simulink library "xbsIndex_r4"  (Simulink 7.1)
PreLoadFcn:
  | warning('off','MATLAB:mex:deprecatedExtension');xlmeta;com.xilinx.sysgen.util.StrategyUtil.loadAllStrategyNames();
values from neighbouring files (symbols this model uses):
  a = xpath.evaluate('//pre:DocumentInfo/pre:Document',x,javax.xml.xpath.XPathConstants.NODESET)    [xlDoc.m]
  n = xpath.evaluate(['//pre:DocumentInfo/pre:Document[@title="'  title                            '"]'],root_elem,javax.xml.xpath.XPathConstants.NODE)    [xlDoc.m]
undefined symbols (not defined in the file or in its folder): gcbh, sim_pause, simulink_period, xlBlockLoadCallback, xlipgetpartsetting, xlRegisterHandles, xlUpdateSgTokenIconStats
libraries: xbsIndex_r4 x18, xbsCopyrightNotice_r4 x1, simulink x1
(part 9 of 9)

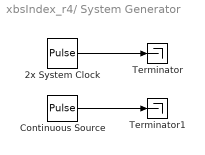
== system xbsIndex_r4/ System Generator ==
  2x System Clock : DiscretePulseGenerator  SampleTime=simulink_period
  Continuous Source : DiscretePulseGenerator  PulseType=Time based  Period=2*simulink_period  PulseWidth=50
  Terminator : Terminator
  Terminator1 : Terminator
  wires:
  Continuous Source/1 -> Terminator1/1
  2x System Clock/1 -> Terminator/1

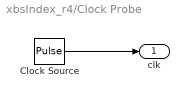
== system xbsIndex_r4/Clock Probe ==
  Clock Source : DiscretePulseGenerator  PhaseDelay=2  SampleTime=(simulink_period/2)
  clk : Outport  OutDataType=sfix(16)  OutScaling=2^0
  wires:
  Clock Source/1 -> clk/1

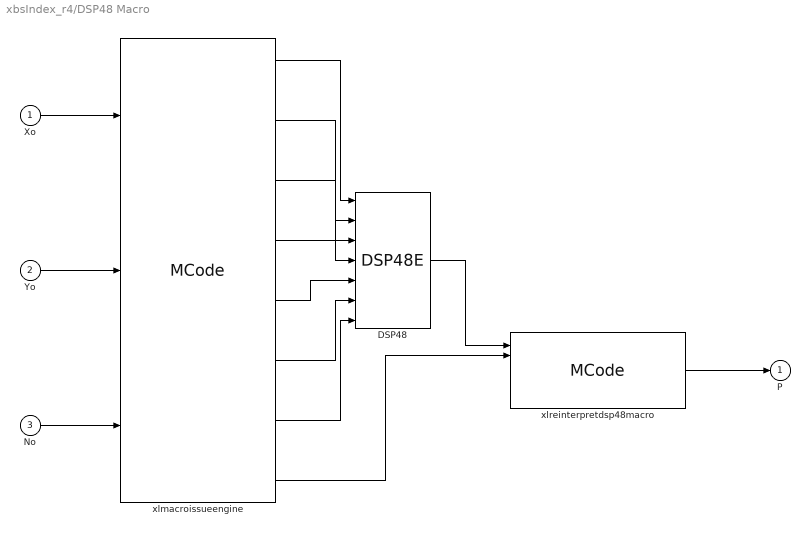
== system xbsIndex_r4/DSP48 Macro ==
  Xo : Inport  OutDataType=sfix(16)  OutScaling=2^0
  Yo : Inport  Port=2  OutDataType=sfix(16)  OutScaling=2^0
  No : Inport  Port=3  OutDataType=sfix(16)  OutScaling=2^0
  DSP48 : xbsIndex_r4/DSP48E  use_a=Direct from A Port  use_b=Direct from B Port  reset_preg=off  pattern_from_creg=on  pattern='000000000000'  mask_from_creg=on  pattern_mask='000000000000'  sel_rounding_mask=Select mask  use_op=off  use_creg=on  rst_all=off  en_all=off  use_pcin=off  use_carrycascin=off  use_multsignin=off  use_carryout=off  use_patterndetect=off  use_patternbdetect=off  use_overflow=off  use_underflow=off  use_acout=off  use_bcout=off  use_pcout=off  use_multsignout=off  use_carrycascout=off  pipeline_a=1  pipeline_b=1  pipeline_acout=1  pipeline_bcout=1  pipeline_c=on  pipeline_p=on  pipeline_mult=on  pipeline_opmode=on  pipeline_alumode=on  pipeline_carryin=on  pipeline_carryinsel=on  rst_a=off  rst_b=off  rst_c=off  rst_mult=off  rst_p=off  rst_carry_in=off  rst_alumode=off  rst_ctrl=off  en_a1=off  en_a2=off  en_b1=off  en_b2=off  en_c=off  en_mult=off  en_p=off  en_carry_in=off  en_alumode=off  en_multcarryin=off  en_ctrl=off  use_synth_model=off  addsub_mode=ONE48  xl_useadderonly=off  block_type=dsp48e
  xlmacroissueengine : xbsIndex_r4/MCode  mfname=xlissue_engine_v5  explicit_period=off  period=1  dbl_ovrd=off  enable_stdout=off  enable_debug=off  suppress_output=on  defparams={'id_a1', 0,'id_a2', 0,'id_a3', 0,'id_a4', 0,'id_a5', 0,'id_a6', 0,'id_a7', 0,'id_b1', 0,'id_b2', 0,'id_b3', 0,'id_b4', 0,'id_b5', 0,'id_b6', 0,'id_b7', 0,'id_c1', 0,'id_c2', 0,'id_c3', 0,'id_c4', 0,'id_c5', 0,'id_c6', 0,'id_c7', 0,'op_const0',53,'op_const1', 0,'op_const2', 0,'op_const3', 0,'op_const4', 0,'op_const5', 0,'op_const6', 0,'op_const7', 0,'alumode_const0',0,'alumode_const1', 0,'alumode_const2', 0,'alumode_const3', 0,'alumode_const4', 0,'alumode_const5', 0,'alumode_const6', 0,'alumode_const7', 0,'carry_in_sel0',0,'carry_in_sel1', 0,'carry_in_sel2', 0,'carry_in_sel3', 0,'carry_in_sel4', 0,'carry_in_sel5', 0,'carry_in_sel6', 0,'carry_in_sel7', 0,'external_cin0', 0,'external_cin1', 0,'external_cin2', 0,'external_cin3', 0,'external_cin4', 0,'external_cin5', 0,'external_cin6', 0,'external_cin7', 0,'reg_a',0,'reg_b',0,'reg_c',0,'reg_op',0,'mode0', 1,'mode1', 0,'mode2', 0,'mode3', 0,'mode4', 0,'mode5', 0,'mode6', 0,'mode7', 0,'ce_all',true,'use_ce_all',false,'sel',0,'rst_all',false,'use_rst_all',false,'cinused',false,'ninstr',1}  hide_port_list={}  block_type=mcode
      settings: xl_area=[0, 0, 0, 0, 0, 0, 0]
  xlreinterpretdsp48macro : xbsIndex_r4/MCode  mfname=xlreinterpretdsp48macro  explicit_period=off  period=1  dbl_ovrd=off  enable_stdout=off  enable_debug=off  suppress_output=off  defparams={'full',precision,'n_bits',n_bits,'bin_pt',bin_pt,'arith_type',arith_type}  hide_port_list={}  block_type=mcode
      settings: xl_area=[0, 0, 0, 0, 0, 0, 0]
  P : Outport  OutDataType=sfix(16)  OutScaling=2^0
  wires:
  xlreinterpretdsp48macro/1 -> P/1
  DSP48/1 -> xlreinterpretdsp48macro/1
  xlmacroissueengine/8 -> xlreinterpretdsp48macro/2
  xlmacroissueengine/7 -> DSP48/7
  xlmacroissueengine/6 -> DSP48/6
  xlmacroissueengine/5 -> DSP48/5
  xlmacroissueengine/4 -> DSP48/4
  xlmacroissueengine/3 -> DSP48/3
  xlmacroissueengine/2 -> DSP48/2
  xlmacroissueengine/1 -> DSP48/1
  No/1 -> xlmacroissueengine/3
  Yo/1 -> xlmacroissueengine/2
  Xo/1 -> xlmacroissueengine/1

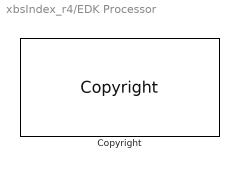
== system xbsIndex_r4/EDK Processor ==
  Copyright : xbsCopyrightNotice_r4/Copyright  copyrighttext="Copyright (c) 2011  by  Xilinx, Inc. All rights reserved.<br><br>This file contains proprietary, confidential information of Xilinx, Inc., is distributed under license from Xilinx, Inc., and may be used, copied and/or disclosed only pursuant to the terms of a valid license agreement with Xilinx, Inc. Xilinx hereby grants you a license to use this file solely for design, simulation, implementation and creation of design files limited to Xilinx devices or technologies. Use with non-Xilinx devices or technologies is expressly prohibited and immediately terminates your license unless covered by a separate agreement.<br><br>Xilinx is providing this design, code, or information \"as-is\" solely for use in developing programs and solutions for Xilinx devices, with no obligation on the part of Xilinx to provide support. By providing this design, code, or information as one possible implementation of this feature, application or standard, Xilinx is making no representation that this implementation is free from any claims of infringement. You are responsible for obtaining any rights you may require for your implementation. Xilinx expressly disclaims any warranty whatsoever with respect to the adequacy of the implementation, including but not limited to any warranties or representations that this implementation is free from claims of infringement, implied warranties of merchantability or fitness for a particular purpose.<br><br>Xilinx products are not intended for use in life support appliances, devices, or systems. Use in such applications is expressly prohibited.<br><br>Any modifications that are made to the Source Code are done at the user's sole risk and will be unsupported.<br><br>This copyright and support notice must be retained as part of this text at all times. (c) Copyright 1995-2011 Xilinx, Inc. All rights reserved."  block_type=copyright
      settings: block_version=10.1.3
      settings: infoedit=|
      | Copyright(C) 2008 by  Xilinx, Inc. All rights reserved.<br>
      | <br>
      | This file contains proprietary, confidential information of Xilinx, Inc., is distributed under license
      | from Xilinx, Inc., and may be used, copied and/or disclosed only pursuant to the terms of a valid license
      | agreement with Xilinx, Inc. Xilinx hereby grants you a license to use this file solely for design,
      | simulation, implementation and creation of design files limited to Xilinx devices or technologies. Use
      | with non-Xilinx devices or technologies is expressly prohibited and immediately terminates your license
      | unless covered by a separate agreement.<br>
      | <br>
      | Xilinx is providing this design, code, or information "as-is" solely for use in developing programs and
      | solutions for Xilinx devices, with no obligation on the part of Xilinx to provide support. By providing
      | this design, code, or information as one possible implementation of this feature, application or standard,
      | Xilinx is making no representation that this implementation is free from any claims of infringement. You
      | are responsible for obtaining any rights you may require for your implementation. Xilinx expressly disclaims
      | any warranty whatsoever with respect to the adequacy of the implementation, including but not limited to any
      | warranties or representations that this implementation is free from claims of infringement, implied warranties
      | of merchantability or fitness for a particular purpose.<br>
      | <br>
      | Xilinx products are not intended for use in life support appliances, devices, or systems. Use in such
      | applications is expressly prohibited.<br>
      | <br>
      | Any modifications that are made to the Source Code are done at the user's sole risk and will be unsupported.<br>
      | <br>
      | This copyright and support notice must be retained as part of this text at all times.
      | (c) Copyright 1995-2008 Xilinx, Inc. All rights reserved.

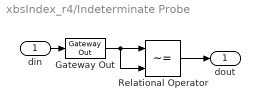
== system xbsIndex_r4/Indeterminate Probe ==
  din : Inport  OutDataType=sfix(16)  OutScaling=2^0
  Gateway Out : xbsIndex_r4/Gateway Out  inherit_from_input=off  hdl_port=off  timing_constraint=None  locs_specified=off  LOCs={}  UseAsDAC=off  DACChannel='1'  block_type=gatewayout
      settings: infoedit="Gateway out block.  Converts Xilinx fixed point inputs into ouputs of type Simulink integer, double, or fixed point.<P><P>Hardware notes:  In hardware these blocks become top level output ports or are discarded, depending on how they are configured."  block_version=9.2-dev
  Relational Operator : RelationalOperator  Operator=~=  InputSameDT=on
  dout : Outport  OutDataType=sfix(16)  OutScaling=2^0
  wires:
  Gateway Out/1 -> Relational Operator/1, Relational Operator/2
  Relational Operator/1 -> dout/1
  din/1 -> Gateway Out/1

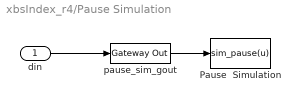
== system xbsIndex_r4/Pause Simulation ==
  din : Inport  OutDataType=sfix(16)  OutScaling=2^0
  Pause  Simulation : MATLABFcn  Priority=1000  MATLABFcn=sim_pause(u)  OutputDimensions=0  Output1D=off
  pause_sim_gout : xbsIndex_r4/Gateway Out  inherit_from_input=off  hdl_port=off  timing_constraint=None  locs_specified=off  LOCs={}  UseAsDAC=off  DACChannel='1'  block_type=gatewayout
      settings: infoedit="Gateway out block.  Converts Xilinx fixed point inputs into ouputs of type Simulink integer, double, or fixed point.<br><br>Hardware notes:  In hardware these blocks become top level output ports or are discarded, depending on how they are configured."  block_version=11.3
  wires:
  pause_sim_gout/1 -> Pause  Simulation/1
  din/1 -> pause_sim_gout/1

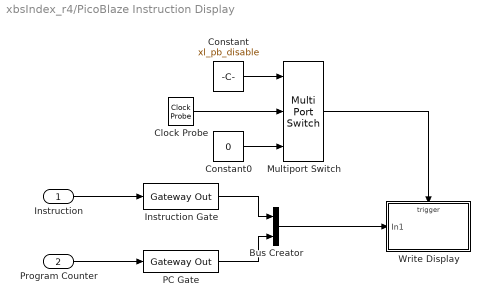
== system xbsIndex_r4/PicoBlaze Instruction Display ==
  Instruction : Inport  OutDataType=sfix(16)  OutScaling=2^0
  Program Counter : Inport  Port=2  OutDataType=sfix(16)  OutScaling=2^0
  Bus Creator : BusCreator  Inputs=2
  Clock Probe : xbsIndex_r4/Clock Probe  SystemSampleTime=-1  block_type=clkprobe
      settings: infoedit="Clock probe.  Produces an output of type double that mirrors the hardware system clock.<P><P>Hardware notes:  This block is ignored when hardware is generated."  block_version=9.1-dev2
  Constant : Constant  Value=xl_pb_disable  OutDataType=sfix(16)  OutScaling=2^0
  Constant0 : Constant  Value=0  OutDataType=sfix(16)  OutScaling=2^0
  Instruction Gate : xbsIndex_r4/Gateway Out  inherit_from_input=off  hdl_port=off  timing_constraint=None  locs_specified=off  LOCs={}  UseAsDAC=off  DACChannel='1'  block_type=gatewayout
      settings: infoedit="Gateway out block.  Converts Xilinx fixed point inputs into ouputs of type Simulink integer, double, or fixed point.<P><P>Hardware notes:  In hardware these blocks become top level output ports or are discarded, depending on how they are configured."  xl_area=[0, 0, 0, 0, 0, 0, 0]  block_version=9.1-dev2
  Multiport Switch : MultiPortSwitch  Inputs=2  zeroidx=on  SaturateOnIntegerOverflow=on
  PC Gate : xbsIndex_r4/Gateway Out  inherit_from_input=off  hdl_port=off  timing_constraint=None  locs_specified=off  LOCs={}  UseAsDAC=off  DACChannel='1'  block_type=gatewayout
      settings: infoedit="Gateway out block.  Converts Xilinx fixed point inputs into ouputs of type Simulink integer, double, or fixed point.<P><P>Hardware notes:  In hardware these blocks become top level output ports or are discarded, depending on how they are configured."  xl_area=[0, 0, 0, 0, 0, 0, 0]  block_version=9.1-dev2
  Write Display : Subsystem  AncestorBlock=xbsIndex_r4/PicoBlaze Instruction Display/Write Display  mask{xl_pb_inst=LOAD sC, 12, xl_pb_pc=17, xl_pb_version=xl_pb_version}
      mask prompts: xl_pb_version "PicoBlaze Version"
  wires:
  Constant0/1 -> Multiport Switch/3
  Clock Probe/1 -> Multiport Switch/2
  Multiport Switch/1 -> Write Display/Trigger
  Constant/1 -> Multiport Switch/1
  Instruction/1 -> Instruction Gate/1
  Program Counter/1 -> PC Gate/1
  Instruction Gate/1 -> Bus Creator/1
  PC Gate/1 -> Bus Creator/2
  Bus Creator/1 -> Write Display/1(In1)

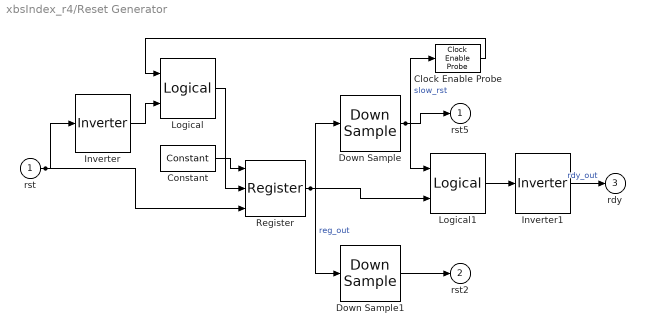
== system xbsIndex_r4/Reset Generator ==
  rst : Inport
  Clock Enable Probe : xbsIndex_r4/Clock Enable Probe  inherit_constraints=on  block_type=ceprobe
      settings: infoedit="Clock enable extractor.  Produces a Boolean output that mirrors the hardware clock enable associated with the input sample rate.<br><br>Hardware notes: in hardware this block costs nothing."
  Constant : xbsIndex_r4/Constant  const=1  gui_display_data_type=Fixed-point  arith_type=Boolean  n_bits=1  bin_pt=0  preci_type=Single  exp_width=8  frac_width=24  explicit_period=off  period=1  equ=P=C  opselect=C  inp2=PCIN>>17  opr=+  inp1=P  carry=CIN  dbl_ovrd=off  block_type=constant
  Down Sample : xbsIndex_r4/Down Sample  sample_ratio=5  sample_phase="Last Value of Frame  (most efficient)"  en=off  latency=1  dbl_ovrd=off  block_type=dsamp
  Down Sample1 : xbsIndex_r4/Down Sample  sample_ratio=2  sample_phase="Last Value of Frame  (most efficient)"  en=off  latency=3  dbl_ovrd=off  block_type=dsamp
  Inverter : xbsIndex_r4/Inverter  en=off  latency=0  dbl_ovrd=off  block_type=inv
  Inverter1 : xbsIndex_r4/Inverter  en=off  latency=0  dbl_ovrd=off  block_type=inv
  Logical : xbsIndex_r4/Logical  logical_function=AND  inputs=2  en=off  latency=0  precision=Full  arith_type=Unsigned  n_bits=16  bin_pt=0  align_bp=on  dbl_ovrd=off  block_type=logical
  Logical1 : xbsIndex_r4/Logical  logical_function=OR  inputs=2  en=off  latency=0  precision=Full  arith_type=Unsigned  n_bits=16  bin_pt=0  align_bp=on  dbl_ovrd=off  block_type=logical
  Register : xbsIndex_r4/Register  init=0  rst=on  en=on  dbl_ovrd=off  block_type=register
  rst5 : Outport
  rst2 : Outport  Port=2
  rdy : Outport  Port=3
  wires:
  Down Sample/1 -> rst5/1, Logical1/1, Clock Enable Probe/1  "slow_rst"
  rst/1 -> Register/3, Inverter/1
  Register/1 -> Down Sample1/1, Logical1/2, Down Sample/1  "reg_out"
  Inverter1/1 -> rdy/1  "rdy_out"
  Down Sample1/1 -> rst2/1
  Logical1/1 -> Inverter1/1
  Logical/1 -> Register/2
  Constant/1 -> Register/1
  Inverter/1 -> Logical/2
  Clock Enable Probe/1 -> Logical/1

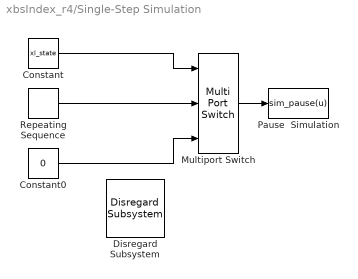
== system xbsIndex_r4/Single-Step Simulation ==
  Constant : Constant  Value=xl_state  OutDataType=sfix(16)  OutScaling=2^0
  Constant0 : Constant  Value=0  OutDataType=sfix(16)  OutScaling=2^0
  Disregard Subsystem : xbsIndex_r4/Disregard Subsystem  Tag=discardX  block_type=disregard
      settings: infoedit="Place this block into any subsystem of a model to indicate that you do not wish System Generator to generate any hardware components for the subsystem.  This block can be used in combination with the Simulation Multiplexer block to build alternative simulation models for a portion of a design (e.g. to provide a simulation model for a black box)."  block_version=11.4
  Multiport Switch : MultiPortSwitch  Inputs=2  zeroidx=on  SaturateOnIntegerOverflow=on
  Pause  Simulation : MATLABFcn  Priority=1000  MATLABFcn=sim_pause(u)  OutputDimensions=0  Output1D=off
  Repeating Sequence : simulink/Sources/Repeating Sequence  SystemSampleTime=-1  rep_seq_t=[0 1]  rep_seq_y=[1 1]
  wires:
  Repeating Sequence/1 -> Multiport Switch/2
  Multiport Switch/1 -> Pause  Simulation/1
  Constant0/1 -> Multiport Switch/3
  Constant/1 -> Multiport Switch/1

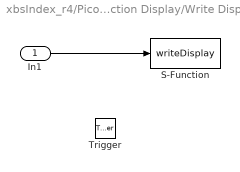
== system xbsIndex_r4/PicoBlaze Instruction Display/Write Display ==
  In1 : Inport  OutDataType=sfix(16)  OutScaling=2^0
  Trigger : TriggerPort  ZeroCross=off
  S-Function : S-Function  FunctionName=writeDisplay  Parameters=xl_pb_version  EnableBusSupport=off  mask(Write Display.){sysname=PBDemo_PicoBlaze__Instruction_Display, xl_pb_version=xl_pb_version}
      mask prompts: sysname "System Name"; xl_pb_version "PicoBlaze Version"
      mask help: Write Display. Writes the instruction and program counter to the display block.
  wires:
  In1/1 -> S-Function/1
